simulink model "Parallel4"  (Simulink 8.7)
settings: Solver=ode45  StartTime=0.0  StopTime=10.0  RelTol=1e-3
settings Model: Creator=scaife  LastModifiedBy=bourbouh  ExtModeAutoUpdateStatusClock=off
settings DataIOCC: SignalLoggingSaveFormat=ModelDataLogs  SignalLoggingName=sigsOut
settings DebuggingCC: SaveWithParameterizedLinksMsg=none  SignalResolutionControl=TryResolveAllWithWarning  MultiTaskDSMMsg=warning  MultiTaskCondExecSysMsg=none
settings HardwareCC: TargetUnknown=on
settings SFSimCC: SimParseCustomCode=off
settings GRTTargetCC: CombineOutputUpdateFcns=off  GRTInterface=on

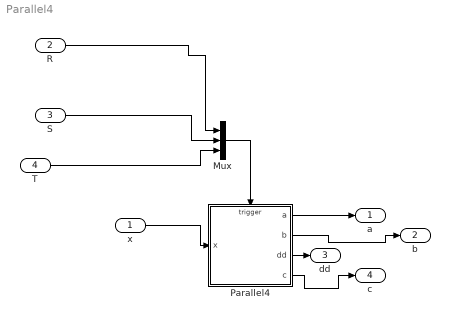
== system Parallel4 ==
  x : Inport
  R : Inport  Port=2
  S : Inport  Port=3
  T : Inport  Port=4
  Mux : Mux  Inputs=3
  Parallel4 : Stateflow chart  TreatAsAtomicUnit=on
  a : Outport
  b : Outport  Port=2
  dd : Outport  Port=3
  c : Outport  Port=4
  wires:
  Mux/1 -> Parallel4/Trigger
  x/1 -> Parallel4/1(x)
  R/1 -> Mux/1
  S/1 -> Mux/2
  T/1 -> Mux/3
  Parallel4/1(a) -> a/1
  Parallel4/2(b) -> b/1
  Parallel4/3(dd) -> dd/1
  Parallel4/4(c) -> c/1

== stateflow chart Parallel4 ==
  state A [parallel]
    settings: executionOrder=1
    state A1
      state A1a/
        en:a=x+1
      state A1b/
        en:a=x+2
      (default) -> A1a
      A1a -> A1b : S
      A1b -> A1a : R
    state A2
      state A2a/
        en:a=x+3
      state A2b/
        en:a=x+4
      (default) -> A2a
      A2a -> A2b : S
      A2b -> A2a [order 2] : R
    (default) -> A1
    A1 -> A2 : T
    A2 -> A1 : T
  state B [parallel]
    settings: executionOrder=2
    state B2
      state B2a/
        en:b=a+7
      state B2b/
        en:b=a+8
      (default) -> B2a
      B2a -> B2b : S
      B2b -> B2a : R
    state B1
      state B1a/
        en:b=a+5
      state B1b/
        en:b=a+6
      (default) -> B1a
      B1a -> B1b : S
      B1b -> B1a : R
    (default) -> B1
    B1 -> B2 : T
    B2 -> B1 : T
  state CD [parallel]
    settings: executionOrder=3
    state C [parallel]
      settings: executionOrder=1
      state C2
        state C2a/
          en:c=b+3
        state C2b/
          en:c=b+4
        (default) -> C2a
        C2a -> C2b : S
        C2b -> C2a : R
      state C1
        state C1a/
          en:c=b+1
        state C1b/
          en:c=b+2
        (default) -> C1a
        C1a -> C1b : S
        C1b -> C1a : R
      (default) -> C1
      C1 -> C2 : T
      C2 -> C1 : T
    state D [parallel]
      settings: executionOrder=2
      state D2
        state D2a/
          en:dd=c+7
        state D2b/
          en:dd=c+8
        (default) -> D2a
        D2a -> D2b : S
        D2b -> D2a : R
      state D1
        state D1a/
          en:dd=c+5
        state D1b/
          en:dd=c+6
        (default) -> D1a
        D1a -> D1b : S
        D1b -> D1a : R
      (default) -> D1
      D1 -> D2 : T
      D2 -> D1 : T
  A2b -> C2a [order 1] : S
  data: a output int32; b output int32; dd output int32; c output int32; x input int32
  events: R input EITHER_EDGE_EVENT; S input EITHER_EDGE_EVENT; T input EITHER_EDGE_EVENT
